simulink model "Radar_Acc_ExtSen_CS9_23Apr"  (Simulink 8.5)
settings: Solver=ode45  StartTime=0  StopTime=100  RelTol=1e-3
values from neighbouring files (symbols this model uses):
  A = block.DialogPrm(16).Data    [mscontroller.m]    (also in mscontrolleracc_23Apr.m = [A;A1]; mscontrolleracc_baru.m; msinitctrl_20Feb.m = [E;H]; msinitctrl_23Apr.m = [E;H])
  a1 = [0.9955446021 3.65450620681e-05 0.013568706589 -0.00380977778976 -3.27390170636e-05 0.999991079318 -0.00155091076214 -8.8453715174e-05 -0.00027528689777 -6.68106743051e-06 1.00030076916 -0.000255683846088 ... (16 elements, 4x4)]    [Modeldua.mat]    (also in Modeldua_baru.mat = [0.9955446021 3.65450625101e-05 0.013568706589 -0.0038097777; identifikasi12Feb.m = th1(1:nstate,:)'; mscontroller.m = block.DialogPrm(17).Data; mscontrolleracc_23Apr.m = block.DialogPrm(17).Data)
  b1 = [-0.432091842363  -0.00101247649361; 0.0169326124942  -2.68146969304e-05; 0.509251329378  -0.00874577361681; -0.418009574499  -0.00119052382537]    [Modeldua.mat]    (also in Modeldua_baru.mat = [-0.432091842361  -0.00101247649364; 0.0169326124949  -2.681; identifikasi12Feb.m = th1(nstate+1:nstate+ni,:)'; mscontroller.m = block.DialogPrm(18).Data; mscontrolleracc_23Apr.m = block.DialogPrm(18).Data)
  c1 = [-1.32625806166  0.301027938745  -0.000253507279411  1.29303056173; -2.69120099418  0.955277024985  0.0214166883856  2.84139544918]    [Modeldua.mat]    (also in Modeldua_baru.mat = [-1.32625824559  0.301027923905  -0.000253508427373  1.29303; identifikasi12Feb.m = th11(1:nstate,:)'; mscontroller.m = block.DialogPrm(19).Data; mscontrolleracc_23Apr.m = block.DialogPrm(19).Data)
  d1 = [-35.3143443825  0.732623315171; -6.47787947029  -0.0810858836178]    [Modeldua.mat]    (also in Modeldua_baru.mat = [-35.3143062638  0.732622901766; -6.47780862608  -0.08108666; identifikasi12Feb.m = th11(nstate+1:nstate+ni,:)'; mscontroller.m = block.DialogPrm(20).Data; mscontrolleracc_23Apr.m = block.DialogPrm(20).Data)
  delta = block.DialogPrm(9).Data    [mscontroller.m]    (also in mscontrolleracc_23Apr.m; mscontrolleracc_baru.m; msinitctrl_20Feb.m = []; msinitctrl_23Apr.m = [])
  ds = 0.5    [msinitctrl_20Feb.m]    (also in msinitctrl_23Apr.m; msref.m = block.DialogPrm(2).Data; msrefacc.m = block.DialogPrm(2).Data; msrefacc_23Apr.m = block.DialogPrm(2).Data)
  f = block.DialogPrm(5).Data    [mscontroller.m]    (also in mscontrolleracc_23Apr.m; mscontrolleracc_baru.m)
  gamma = block.DialogPrm(8).Data    [mscontroller.m]    (also in mscontrolleracc_23Apr.m; mscontrolleracc_baru.m; msinitctrl_20Feb.m = temp*temp2; msinitctrl_23Apr.m = temp*temp2)
  H = block.DialogPrm(6).Data    [mscontroller.m]    (also in mscontrolleracc_23Apr.m; mscontrolleracc_baru.m; msinitctrl_20Feb.m = zeros(2*ni*m,ni*m); msinitctrl_23Apr.m = zeros(2*ni*m,ni*m))
  kx1 = [0.373805533072 -0.00539111413138 -0.939878164031 0.330283524969]    [Modeldua.mat]    (also in Modeldua_baru.mat = [0.373805533072 -0.0053911141315 -0.939878164031 0.330283524; identifikasi12Feb.m = th1(nstate+ni+1,:)'; mscontroller.m = block.DialogPrm(21).Data; mscontrolleracc_23Apr.m = block.DialogPrm(21).Data)
  ky1 = [151.759221905 176.849822393]    [Modeldua.mat]    (also in Modeldua_baru.mat = [151.759227597 176.849976774]; identifikasi12Feb.m = th11(nstate+ni+1,:)'; mscontroller.m = block.DialogPrm(22).Data; mscontrolleracc_23Apr.m = block.DialogPrm(22).Data)
  L = 3.048    [msinitctrl_20Feb.m]    (also in msinitctrl_23Apr.m; msref.m = block.DialogPrm(3).Data; msrefacc.m = block.DialogPrm(3).Data; msrefacc_23Apr.m = block.DialogPrm(3).Data)
  ni = 2    [Modeldua.mat]    (also in Modeldua_baru.mat; identifikasi12Feb.m; mscontroller.m = block.DialogPrm(3).Data; mscontrolleracc_23Apr.m = block.DialogPrm(3).Data)
  no = 2    [Modeldua.mat]    (also in Modeldua_baru.mat; identifikasi12Feb.m; mscontroller.m = block.DialogPrm(2).Data; mscontrolleracc_23Apr.m = block.DialogPrm(2).Data)
  p = block.DialogPrm(1).Data    [mscontroller.m]    (also in mscontrolleracc_23Apr.m; mscontrolleracc_baru.m; msinitctrl_20Feb.m = 5; msinitctrl_23Apr.m = 5)
  phi = block.DialogPrm(10).Data    [mscontroller.m]    (also in mscontrolleracc_23Apr.m; mscontrolleracc_baru.m; msinitctrl_20Feb.m = temp*temp4; msinitctrl_23Apr.m = temp*temp4)
  psi = block.DialogPrm(7).Data    [mscontroller.m]    (also in mscontrolleracc_23Apr.m; mscontrolleracc_baru.m; msinitctrl_20Feb.m = temp*temp1; msinitctrl_23Apr.m = temp*temp1)
  Q = block.DialogPrm(14).Data    [mscontroller.m]    (also in mscontrolleracc_23Apr.m; mscontrolleracc_baru.m; msinitctrl_20Feb.m = q*eye(p*no); msinitctrl_23Apr.m = q*eye(p*no))
  R = block.DialogPrm(15).Data    [mscontroller.m]    (also in mscontrolleracc_23Apr.m; mscontrolleracc_baru.m; msinitctrl_20Feb.m = r*eye(m*ni); msinitctrl_23Apr.m = r*eye(m*ni))
  sudut_sensor = 10    [msinitctrl_20Feb.m]    (also in msinitctrl_23Apr.m; msref.m = block.DialogPrm(4).Data; msrefacc.m = block.DialogPrm(4).Data; msrefacc_23Apr.m = block.DialogPrm(4).Data)
  tau = 1.5    [msinitctrl_20Feb.m]    (also in msinitctrl_23Apr.m; msref.m = block.DialogPrm(1).Data; msrefacc.m = block.DialogPrm(1).Data; msrefacc_23Apr.m = block.DialogPrm(1).Data)
  th = block.DialogPrm(12).Data    [mscontroller.m]    (also in mscontrolleracc_23Apr.m; mscontrolleracc_baru.m; msinitctrl_20Feb.m = temp*temp3; msinitctrl_23Apr.m = temp*temp3)
  umax = block.DialogPrm(24).Data    [mscontroller.m]    (also in mscontrolleracc_23Apr.m; mscontrolleracc_baru.m; msinitctrl_20Feb.m = [umax1;umax2]; msinitctrl_23Apr.m = [umax1;umax2])
  umin = block.DialogPrm(23).Data    [mscontroller.m]    (also in mscontrolleracc_23Apr.m; mscontrolleracc_baru.m; msinitctrl_20Feb.m = [umin1;umin2]; msinitctrl_23Apr.m = [umin1;umin2])
  upsilon = block.DialogPrm(13).Data    [mscontroller.m]    (also in mscontrolleracc_23Apr.m; mscontrolleracc_baru.m; msinitctrl_20Feb.m = []; msinitctrl_23Apr.m = [])
  xi = block.DialogPrm(11).Data    [mscontroller.m]    (also in mscontrolleracc_23Apr.m; mscontrolleracc_baru.m; msinitctrl_20Feb.m = []; msinitctrl_23Apr.m = [])
libraries: Solver_SF x2, simulink x1
settings Model: Creator=dhall  LastModifiedBy=Mastereal  ExtModeTrigMode=oneshot  ExtModeArmWhenConnect=off
settings DataIOCC: LimitDataPoints=off  SignalLoggingName=sigsOut
settings OptimizationCC: BooleanDataType=off  ExpressionDepthLimit=128  LocalBlockOutputs=off  InitFltsAndDblsToZero=on
settings DebuggingCC: SaveWithParameterizedLinksMsg=none  SignalResolutionControl=TryResolveAllWithWarning  MultiTaskDSMMsg=warning  MultiTaskCondExecSysMsg=none  FcnCallInpInsideContextMsg=UseLocalSettings
settings HardwareCC: TargetUnknown=on
settings GRTTargetCC: TargetFcnLib=ansi_tfl_tmw.mat  CompOptLevelCompliant=off

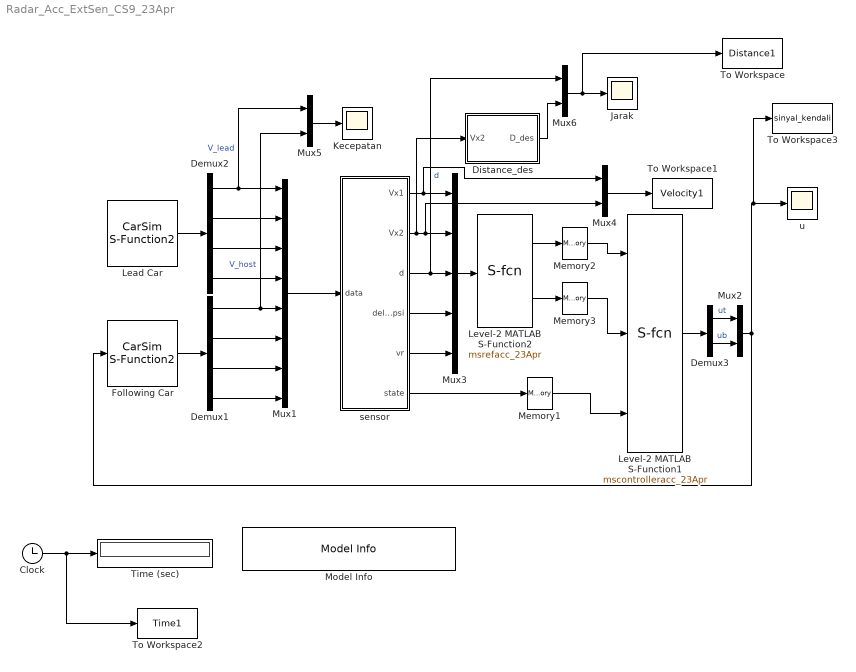
== system Radar_Acc_ExtSen_CS9_23Apr ==
  Clock : Clock
  Demux1 : Demux
  Demux2 : Demux
  Demux3 : Demux  Outputs=2
  Distance_des : MATLAB Function  TreatAsAtomicUnit=on
  Following Car : Solver_SF/CarSim S-Function2  Priority=1  VehicleCode=i_i2  SIMFILE=Radar_Acc_ExtSen_Car_2.sim
      settings: AttributesFormatString=Vehicle Code: %<VehicleCode>
  Jarak : Scope
      settings: TickLabels=on  ShowLegends=on  TimeRange=50  YMin=29  YMax=45  MaxDataPoints=50000  SampleTime=100
  Kecepatan : Scope
      settings: TickLabels=on  ShowLegends=on  TimeRange=50  YMin=59.5  YMax=70.5  MaxDataPoints=50000  SampleTime=100
  Lead Car : Solver_SF/CarSim S-Function2  Priority=1  VehicleCode=i_i  SIMFILE=Radar_Acc_ExtSen_Car_1.sim
      settings: AttributesFormatString=Vehicle Code: %<VehicleCode>
  Level-2 MATLAB S-Function1 : M-S-Function  FunctionName=mscontrolleracc_23Apr  Parameters=p,no,ni,e,f,H,psi,gamma,delta,phi,xi,th,upsilon,Q,R,A,a1,b1,c1,d1,kx1,ky1,umin,umax
  Level-2 MATLAB S-Function2 : M-S-Function  FunctionName=msrefacc_23Apr  Parameters=tau,ds,L,sudut_sensor,ni,p
  Memory1 : Memory
  Memory2 : Memory
  Memory3 : Memory
  Model Info : simulink/Model-Wide Utilities/Model Info  Frame=on  DisplayStringWithTags=Multi Vehicle Run Adaptive Cruise Control Model  HorizontalTextAlignment=Center  LeftAlignmentValue=0.5  SourceBlockDiagram=Radar_Acc_ExtSen_CS9_23Apr  TagMaxNumber=20
  Mux1 : Mux  Inputs=8
  Mux{2,4..6} (4 alike) : Mux  Inputs=2
  Mux3 : Mux  Inputs=5
  Time (sec) : Display
      settings: Format=bank  Decimation=100
  To Workspace : ToWorkspace  VariableName=Distance1  SampleTime=0.001
  To Workspace1 : ToWorkspace  VariableName=Velocity1  SampleTime=0.001
  To Workspace2 : ToWorkspace  VariableName=Time1  SampleTime=0.001
  To Workspace3 : ToWorkspace  VariableName=sinyal_kendali  SampleTime=0.001
  sensor : MATLAB Function  TreatAsAtomicUnit=on
  u : Scope
      settings: TickLabels=on  ShowLegends=on  TimeRange=50  YMin=0.1  YMax=1.2  SaveName=ScopeData2  MaxDataPoints=50000  SampleTime=100
  wires:
  Clock/1 -> To Workspace2/1, Time (sec)/1
  Following Car/1 -> Demux1/1
  Lead Car/1 -> Demux2/1
  Demux2/1 -> Mux1/1, Mux5/1  "V_lead"
  Demux2/2 -> Mux1/2
  Demux2/3 -> Mux1/3
  Demux2/4 -> Mux1/4
  Demux1/1 -> Mux5/2, Mux1/5  "V_host"
  Demux1/2 -> Mux1/6
  Demux1/3 -> Mux1/7
  Demux1/4 -> Mux1/8
  Mux1/1 -> sensor/1(data)
  sensor/1(Vx1) -> Mux4/1, Mux3/1
  sensor/2(Vx2) -> Distance_des/1(Vx2), Mux4/2, Mux3/2
  sensor/3(d) -> Mux6/1, Mux3/3  "d"
  sensor/4(delta_psi) -> Mux3/4
  sensor/5(vr) -> Mux3/5
  Mux3/1 -> Level-2 MATLAB S-Function2/1
  sensor/6(state) -> Memory1/1
  Level-2 MATLAB S-Function1/1 -> Demux3/1
  Demux3/1 -> Mux2/1  "ut"
  Demux3/2 -> Mux2/2  "ub"
  Mux2/1 -> To Workspace3/1, u/1, Following Car/1
  Mux5/1 -> Kecepatan/1
  Mux6/1 -> To Workspace/1, Jarak/1
  Distance_des/1(D_des) -> Mux6/2
  Level-2 MATLAB S-Function2/1 -> Memory2/1
  Level-2 MATLAB S-Function2/2 -> Memory3/1
  Memory2/1 -> Level-2 MATLAB S-Function1/1
  Memory3/1 -> Level-2 MATLAB S-Function1/2
  Memory1/1 -> Level-2 MATLAB S-Function1/3
  Mux4/1 -> To Workspace1/1

== matlab function Distance_des ==
  data: Vx2 input double; D_des output double
function D_des  = fcn(Vx2)
%#codegen
L=3.048; tau=1.5; ds=0.5; sudut_sensor = 10;
D_des = L+ds+tau*(Vx2*(1000/3600));

== matlab function sensor ==
  data: data input double; Vx1 output double; Vx2 output double; d output double; delta_psi output double; vr output double; state output double
function [Vx1,Vx2,d,delta_psi,vr,state] = fcn(data)
%#codegen
%pembagian sinyal
Vx1= data(1);
X1= data(2);
Y1= data(3);
psi1= data(4);
Vx2= data(5);
X2= data(6);
Y2= data(7);
psi2= data(8);

psi2fix = mod(psi2,360);

Xo = X1-X2;
Yo = Y1-Y2;
d = sqrt(Xo^2 + Yo^2);
anglerad = atan(Yo/Xo);
anglesudut = anglerad*(180/pi);
sudut = abs(anglesudut-psi2fix);

suduta = sudut;
sudutb = 360 - sudut;

if sudutb >= 270
   delta_psi = suduta;
else 
    delta_psi = sudutb;
end

vr = Vx2-Vx1;

state = [Vx2;d;delta_psi;vr];
